simulink subsystem "Combustion"  (R2024b)
settings: Solver=VariableStepAuto  StartTime=0.0  StopTime=10.0  RelTol=1e-3
settings Model: Creator=The MathWorks, Inc.  LastModifiedBy=The MathWorks, Inc.

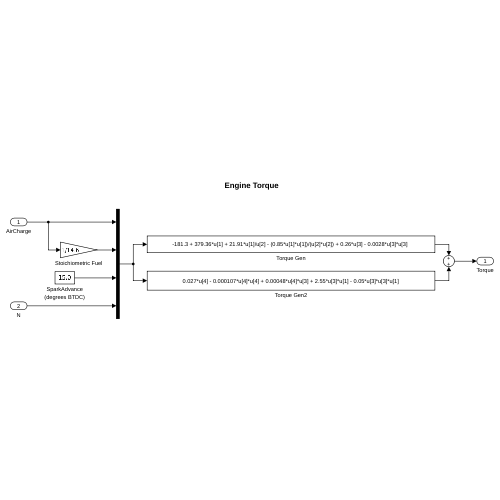
[thumbnail: Simulink's stored preview of the top-level diagram]
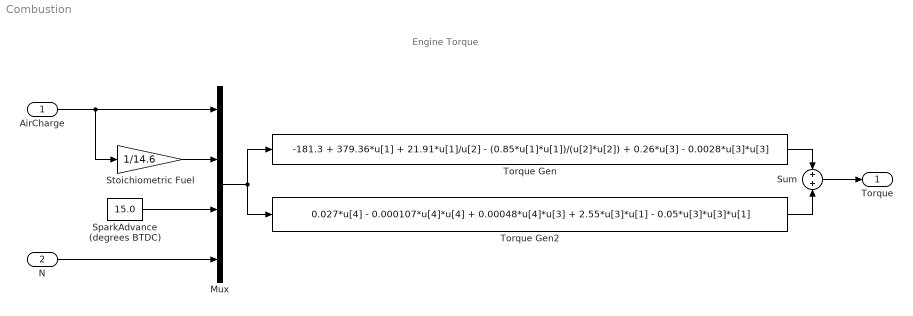
== system Combustion ==
  note: Engine Torque
  AirCharge : Inport
  N : Inport  Port=2
  Mux : Mux
  SparkAdvance (degrees BTDC) : Constant  Value=15.0
  Stoichiometric Fuel : Gain  Gain=1/14.6  SaturateOnIntegerOverflow=on  OutDataTypeStr=Inherit: Same as input  ParamDataTypeStr=Inherit: Same as input
  Sum : Sum  InputSameDT=on  SaturateOnIntegerOverflow=on  OutDataTypeStr=Inherit: Same as first input
  Torque Gen : Fcn  Expr=-181.3 + 379.36*u[1] + 21.91*u[1]/u[2] - (0.85*u[1]*u[1])/(u[2]*u[2]) + 0.26*u[3] - 0.0028*u[3]*u[3]
  Torque Gen2 : Fcn  Expr=0.027*u[4] - 0.000107*u[4]*u[4] + 0.00048*u[4]*u[3] + 2.55*u[3]*u[1] - 0.05*u[3]*u[3]*u[1]
  Torque : Outport  InitialOutput=0  VectorParamsAs1DForOutWhenUnconnected=off
  wires:
  Sum/1 -> Torque/1
  Torque Gen/1 -> Sum/1
  Torque Gen2/1 -> Sum/2
  Mux/1 -> Torque Gen2/1, Torque Gen/1
  AirCharge/1 -> Stoichiometric Fuel/1, Mux/1
  N/1 -> Mux/4
  SparkAdvance (degrees BTDC)/1 -> Mux/3
  Stoichiometric Fuel/1 -> Mux/2
